simulink library "EdgesLibrary"  (R2021a)
settings: Solver=VariableStepAuto  StartTime=0.0  StopTime=10.0  RelTol=1e-3
undefined symbols (not defined in the file): Rk
libraries: $bdroot x11, simulink x5
settings Model: Creator=phill  LastModifiedBy=phill

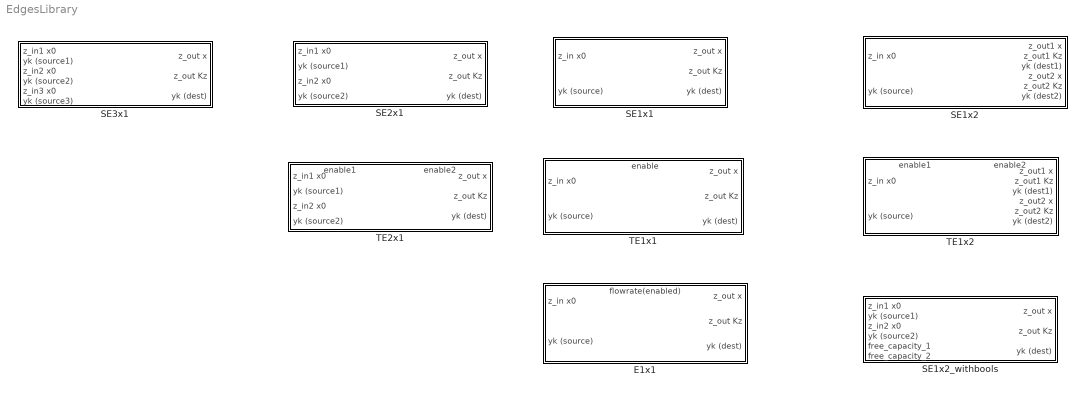
== system EdgesLibrary ==
  E1x1 : Subsystem
      mask help: This block serves to establish a flow between two Street Lane Segments. To archieve this, it connects one source-cell [z_in] to one destination-cell [z_out], and prompts a flow of cars with the flowrate 'flowrate(enabled)' (an input) if and only if there are still cars at the end of [z_out] avaiable AND if the capacity of [z_out] is not yet surpassed, i.e. (z_in x0 > 0 AND z_out Kz > z_out x), otherwise the flow is reduced to 0.
      settings: PortSchema="{\"entries\":[{\"content\":{\"sides\":[{\"content\":{\"connectorIds\":[\"In1\",\"Out2\"]},\"type\":\"ConnectorPlacement.EquallySpacedRectSide\",\"uuid\":\"c2e99070-5232-4a61-a40f-9294101b0b00\"},{\"content\":{\"connectorIds\":[\"In3\",\"In4\",\"Out1\"],\"side\":\"RIGHT\"},\"type\":\"ConnectorPlacement.EquallySpacedRectSide\",\"uuid\":\"7311a175-c780-45f4-b469-43cf69089bcd\"},{\"content\":{\"connectorIds\":[\"In2\"],\"side\":\"TOP\"},\"type\":\"ConnectorPlacement.EquallySpacedRectSide\",\"uuid\":\"52e907de-6c11-4251-aa6b-7e90a209cdcc\"}]},\"type\":\"ConnectorPlacement.EquallySpacedConnector\",\"uuid\":\"2a0e9608-1744-4ca6-8ee9-50c44ff0c1fb\"}],\"packageUris\":[\"http://schema.mathworks.com/mf0/Connector/R2020b\"],\"version\":\"1.0\"}"
      mask Display:
      | image('$imagefile'); % Use "Edit Image" on toolstrip to change.
      | % image('$imagefile');
      | disp('Edge 1x1');
  SE1x1 : Subsystem  mask{Rk=0, slope=2000}
      mask prompts: Rk "Rk (fixed flowrate, used when the flow is enabled)"
      mask help: This block serves to establish a flow between two Street Lane Segments. To archieve this, it connects one source-cell [z_in] to one destination-cell [z_out], and prompts a flow of cars with the rate Rk (Parameter) if and only if there are still cars at the end of [z_out] avaiable and if the capacity of [z_out] is not yet surpassed, i.e. (z_in x0 > 0 AND z_out Kz > z_out x), otherwise the flow is reduced to 0.
      settings: PortSchema="{\"entries\":[{\"content\":{\"sides\":[{\"content\":{\"connectorIds\":[\"In1\",\"Out2\"]},\"type\":\"ConnectorPlacement.EquallySpacedRectSide\",\"uuid\":\"f9c1cf46-46ac-4011-8499-7a2e74fc4a3a\"},{\"content\":{\"connectorIds\":[\"In2\",\"In3\",\"Out1\"],\"side\":\"RIGHT\"},\"type\":\"ConnectorPlacement.EquallySpacedRectSide\",\"uuid\":\"f685a77a-a8b9-4a29-8679-dc3cbf3c2b7f\"},{\"content\":{\"connectorIds\":[],\"side\":\"TOP\"},\"type\":\"ConnectorPlacement.EquallySpacedRectSide\",\"uuid\":\"af8d715a-ddb3-4f5e-8163-596be4e65ef7\"}]},\"type\":\"ConnectorPlacement.EquallySpacedConnector\",\"uuid\":\"ace495d2-b7cd-4153-a555-4989f077c969\"}],\"packageUris\":[\"http://schema.mathworks.com/mf0/Connector/R2020b\"],\"version\":\"1.0\"}"
      mask Display:
      | image('$imagefile'); % Use "Edit Image" on toolstrip to change.
      | % image('$imagefile');
      | disp('Simple Edge 1x1 \n\n');
      | disp(['Rk = ', get_param(gcb,'Rk'),' slope = ', get_param(gcb,'slope')])
  SE1x2 : Subsystem  mask{Rk1=0, Rk2=0}
      mask prompts: Rk1 "Rk (output 1)"; Rk2 "Rk (output 2)"
      settings: PortSchema="{\"entries\":[{\"content\":{\"sides\":[{\"content\":{\"connectorIds\":[\"In1\",\"Out3\"]},\"type\":\"ConnectorPlacement.EquallySpacedRectSide\",\"uuid\":\"58588114-80b7-4cf3-8a8f-92af49331a70\"},{\"content\":{\"connectorIds\":[\"In2\",\"In3\",\"Out1\",\"In4\",\"In5\",\"Out2\"],\"side\":\"RIGHT\"},\"type\":\"ConnectorPlacement.EquallySpacedRectSide\",\"uuid\":\"0e7c0143-84e4-4501-996a-3b666730c0e6\"},{\"content\":{\"connectorIds\":[],\"side\":\"TOP\"},\"type\":\"ConnectorPlacement.EquallySpacedRectSide\",\"uuid\":\"990b873b-8878-4c8e-bdf4-2f621fb88a1c\"}]},\"type\":\"ConnectorPlacement.EquallySpacedConnector\",\"uuid\":\"e53b41a9-82b8-4753-89eb-fe06ea1139d8\"}],\"packageUris\":[\"http://schema.mathworks.com/mf0/Connector/R2020b\"],\"version\":\"1.0\"}"
      mask Display:
      | image('$imagefile'); % Use "Edit Image" on toolstrip to change.
      | % image('$imagefile');
      | disp('Simple Edge 1x2\n\n\n');
      | tRk = get_param(gcb,'Rk1');
      | w1 = get_param(gcb, 'Rk2');
      | disp(['Rk1 = ', tRk, ' | Rk2 =  ', w1])
  SE1x2_withbools : Subsystem  mask{Rk1=Rk, Rk2=Rk}
      mask prompts: Rk1 "Rk (input 1)"; Rk2 "Rk (input 2)"
      settings: PortSchema="{\"entries\":[{\"content\":{\"sides\":[{\"content\":{\"connectorIds\":[\"In1\",\"Out2\",\"In2\",\"Out3\",\"Out4\",\"Out5\"]},\"type\":\"ConnectorPlacement.EquallySpacedRectSide\",\"uuid\":\"eb102e1f-8f68-4819-b192-9ed8ea7965cd\"},{\"content\":{\"connectorIds\":[\"In3\",\"In4\",\"Out1\"],\"side\":\"RIGHT\"},\"type\":\"ConnectorPlacement.EquallySpacedRectSide\",\"uuid\":\"0a8d41cc-2128-49e0-9ce9-20439c8bfca2\"},{\"content\":{\"connectorIds\":[],\"side\":\"TOP\"},\"type\":\"ConnectorPlacement.EquallySpacedRectSide\",\"uuid\":\"ce1e229b-7216-4f3c-b1ef-7720ca51f1c4\"}]},\"type\":\"ConnectorPlacement.EquallySpacedConnector\",\"uuid\":\"c8e8c67c-b38f-484f-95e7-011277152545\"}],\"packageUris\":[\"http://schema.mathworks.com/mf0/Connector/R2020b\"],\"version\":\"1.0\"}"
      mask Display:
      | image('$imagefile'); % Use "Edit Image" on toolstrip to change.
      | disp('Simple Edge 2x1\n\n\n');
      | Rk1 = get_param(gcb,'Rk1');
      | Rk2 = get_param(gcb, 'Rk2');
      | disp(['Rk1 = ', Rk1, ' | Rk2 =  ', Rk2])
  SE2x1 : Subsystem  mask{Rk1=0, Rk2=0}
      mask prompts: Rk1 "Rk (input 1)"; Rk2 "Rk (input 2)"
      settings: PortSchema="{\"entries\":[{\"content\":{\"sides\":[{\"content\":{\"connectorIds\":[\"In1\",\"Out2\",\"In2\",\"Out3\"]},\"type\":\"ConnectorPlacement.EquallySpacedRectSide\",\"uuid\":\"eb102e1f-8f68-4819-b192-9ed8ea7965cd\"},{\"content\":{\"connectorIds\":[\"In3\",\"In4\",\"Out1\"],\"side\":\"RIGHT\"},\"type\":\"ConnectorPlacement.EquallySpacedRectSide\",\"uuid\":\"0a8d41cc-2128-49e0-9ce9-20439c8bfca2\"},{\"content\":{\"connectorIds\":[],\"side\":\"TOP\"},\"type\":\"ConnectorPlacement.EquallySpacedRectSide\",\"uuid\":\"ce1e229b-7216-4f3c-b1ef-7720ca51f1c4\"}]},\"type\":\"ConnectorPlacement.EquallySpacedConnector\",\"uuid\":\"c8e8c67c-b38f-484f-95e7-011277152545\"}],\"packageUris\":[\"http://schema.mathworks.com/mf0/Connector/R2020b\"],\"version\":\"1.0\"}"
      mask Display:
      | image('$imagefile'); % Use "Edit Image" on toolstrip to change.
      | disp('Simple Edge 2x1\n\n\n');
      | Rk1 = get_param(gcb,'Rk1');
      | Rk2 = get_param(gcb, 'Rk2');
      | disp(['Rk1 = ', Rk1, ' | Rk2 =  ', Rk2])
  SE3x1 : Subsystem  mask{Rk1=0, Rk2=0, Rk3=0}
      mask prompts: Rk1 "Rk (input 1)"; Rk2 "Rk (input 2)"; Rk3 "Rk (input 3)"
      settings: PortSchema="{\"entries\":[{\"content\":{\"sides\":[{\"content\":{\"connectorIds\":[\"In1\",\"Out2\",\"In2\",\"Out3\",\"In3\",\"Out4\"]},\"type\":\"ConnectorPlacement.EquallySpacedRectSide\",\"uuid\":\"eb102e1f-8f68-4819-b192-9ed8ea7965cd\"},{\"content\":{\"connectorIds\":[\"In4\",\"In5\",\"Out1\"],\"side\":\"RIGHT\"},\"type\":\"ConnectorPlacement.EquallySpacedRectSide\",\"uuid\":\"0a8d41cc-2128-49e0-9ce9-20439c8bfca2\"},{\"content\":{\"connectorIds\":[],\"side\":\"TOP\"},\"type\":\"ConnectorPlacement.EquallySpacedRectSide\",\"uuid\":\"ce1e229b-7216-4f3c-b1ef-7720ca51f1c4\"}]},\"type\":\"ConnectorPlacement.EquallySpacedConnector\",\"uuid\":\"c8e8c67c-b38f-484f-95e7-011277152545\"}],\"packageUris\":[\"http://schema.mathworks.com/mf0/Connector/R2020b\"],\"version\":\"1.0\"}"
      mask Display:
      | image('$imagefile'); % Use "Edit Image" on toolstrip to change.
      | disp('Simple Edge 3x1\n\n\n');
      | Rk1 = get_param(gcb,'Rk1');
      | Rk2 = get_param(gcb, 'Rk2');
      | Rk3 = get_param(gcb, 'Rk3');
      | disp(['Rk1 = ', Rk1, ' | Rk2 =  ', Rk2, '\n | Rk3 = ', Rk3])
  TE1x1 : Subsystem  mask{Rk=0, slope=2000}
      mask prompts: Rk "Rk (fixed flowrate, used when the flow is enabled)"
      mask help: This block serves to establish a flow between two Street Lane Segments. To archieve this, it connects one source-cell [z_in] to one destination-cell [z_out], and prompts a flow of cars with the rate Rk (Parameter) if and only if there are still cars at the end of [z_out] avaiable AND if the capacity of [z_out] is not yet surpassed, i.e. (z_in x0 > 0 AND z_out Kz > z_out x), AND if the 'enable' input is set to 1, otherwise the flow is reduced to 0.
      settings: PortSchema="{\"entries\":[{\"content\":{\"sides\":[{\"content\":{\"connectorIds\":[\"In1\",\"Out2\"]},\"type\":\"ConnectorPlacement.EquallySpacedRectSide\",\"uuid\":\"c2e99070-5232-4a61-a40f-9294101b0b00\"},{\"content\":{\"connectorIds\":[\"In3\",\"In4\",\"Out1\"],\"side\":\"RIGHT\"},\"type\":\"ConnectorPlacement.EquallySpacedRectSide\",\"uuid\":\"7311a175-c780-45f4-b469-43cf69089bcd\"},{\"content\":{\"connectorIds\":[\"In2\"],\"side\":\"TOP\"},\"type\":\"ConnectorPlacement.EquallySpacedRectSide\",\"uuid\":\"52e907de-6c11-4251-aa6b-7e90a209cdcc\"}]},\"type\":\"ConnectorPlacement.EquallySpacedConnector\",\"uuid\":\"2a0e9608-1744-4ca6-8ee9-50c44ff0c1fb\"}],\"packageUris\":[\"http://schema.mathworks.com/mf0/Connector/R2020b\"],\"version\":\"1.0\"}"
      mask Display:
      | image('$imagefile'); % Use "Edit Image" on toolstrip to change.
      | % image('$imagefile');
      | disp('Toggleable Edge 1x1 \n\n');
      | disp(['Rk = ', get_param(gcb,'Rk'),' slope = ', get_param(gcb,'slope')])
  TE1x2 : Subsystem  mask{Rk1=0, Rk2=0}
      mask prompts: Rk1 "Rk (output 1)"; Rk2 "Rk (output 2)"
      settings: PortSchema="{\"entries\":[{\"content\":{\"sides\":[{\"content\":{\"connectorIds\":[\"In1\",\"Out3\"]},\"type\":\"ConnectorPlacement.EquallySpacedRectSide\",\"uuid\":\"2e9f11d3-65d9-473f-b826-57e0db4d0b8d\"},{\"content\":{\"connectorIds\":[\"In4\",\"In5\",\"Out1\",\"In6\",\"In7\",\"Out2\"],\"side\":\"RIGHT\"},\"type\":\"ConnectorPlacement.EquallySpacedRectSide\",\"uuid\":\"d8eabf6d-fb3a-4c3e-97ce-4f99fedc7242\"},{\"content\":{\"connectorIds\":[\"In2\",\"In3\"],\"side\":\"TOP\"},\"type\":\"ConnectorPlacement.EquallySpacedRectSide\",\"uuid\":\"c1317a9d-7aa4-490c-a27e-f3fa93a0d151\"}]},\"type\":\"ConnectorPlacement.EquallySpacedConnector\",\"uuid\":\"3cd892e4-da09-4624-b831-53c46896b420\"}],\"packageUris\":[\"http://schema.mathworks.com/mf0/Connector/R2020b\"],\"version\":\"1.0\"}"
      mask Display:
      | image('$imagefile'); % Use "Edit Image" on toolstrip to change.
      | disp('Toggleable Edge 1x2 \n\n');
      | Rk1 = get_param(gcb,'Rk1');
      | Rk2 = get_param(gcb, 'Rk2');
      | disp(['Rk1 = ', Rk1, ' | Rk2 =  ', Rk2])
  TE2x1 : Subsystem  mask{Rk1=0, Rk2=0.5}
      mask prompts: Rk1 "Rk (input 1)"; Rk2 "Rk (input 2)"
      settings: PortSchema="{\"entries\":[{\"content\":{\"sides\":[{\"content\":{\"connectorIds\":[\"In1\",\"Out2\",\"In2\",\"Out3\"]},\"type\":\"ConnectorPlacement.EquallySpacedRectSide\",\"uuid\":\"2e9f11d3-65d9-473f-b826-57e0db4d0b8d\"},{\"content\":{\"connectorIds\":[\"In5\",\"In6\",\"Out1\"],\"side\":\"RIGHT\"},\"type\":\"ConnectorPlacement.EquallySpacedRectSide\",\"uuid\":\"d8eabf6d-fb3a-4c3e-97ce-4f99fedc7242\"},{\"content\":{\"connectorIds\":[\"In3\",\"In4\"],\"side\":\"TOP\"},\"type\":\"ConnectorPlacement.EquallySpacedRectSide\",\"uuid\":\"c1317a9d-7aa4-490c-a27e-f3fa93a0d151\"}]},\"type\":\"ConnectorPlacement.EquallySpacedConnector\",\"uuid\":\"3cd892e4-da09-4624-b831-53c46896b420\"}],\"packageUris\":[\"http://schema.mathworks.com/mf0/Connector/R2020b\"],\"version\":\"1.0\"}"
      mask Display:
      | image('$imagefile'); % Use "Edit Image" on toolstrip to change.
      | disp('Toggleable Edge 2x1 \n\n');
      | Rk1 = get_param(gcb,'Rk1');
      | Rk2 = get_param(gcb, 'Rk2');
      | disp(['Rk1 = ', Rk1, ' | Rk2 =  ', Rk2])

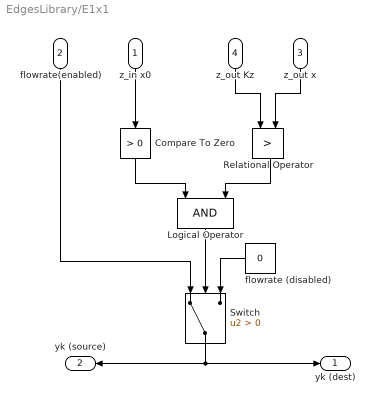
== system EdgesLibrary/E1x1 ==
  z_in x0 : Inport
  flowrate(enabled) : Inport  Port=2
  z_out x : Inport  Port=3
  z_out Kz : Inport  Port=4
  Compare To Zero : simulink/Logic and Bit Operations/Compare To Zero  relop=>  OutDataTypeStr=boolean
  Logical Operator : Logic  Inputs=3  AllPortsSameDT=off  OutDataTypeStr=boolean
  Relational Operator : RelationalOperator  Operator=>  OutDataTypeStr=boolean  RndMeth=Simplest
  Switch : Switch  Criteria=u2 > Threshold
  flowrate (disabled) : Constant  Value=0
  yk (dest) : Outport
  yk (source) : Outport  Port=2
  wires:
  z_out Kz/1 -> Relational Operator/1
  z_out x/1 -> Relational Operator/2
  Logical Operator/1 -> Switch/2
  flowrate(enabled)/1 -> Switch/1
  flowrate (disabled)/1 -> Switch/3
  z_in x0/1 -> Compare To Zero/1
  Compare To Zero/1 -> Logical Operator/1
  Relational Operator/1 -> Logical Operator/3
  Switch/1 -> yk (source)/1, yk (dest)/1

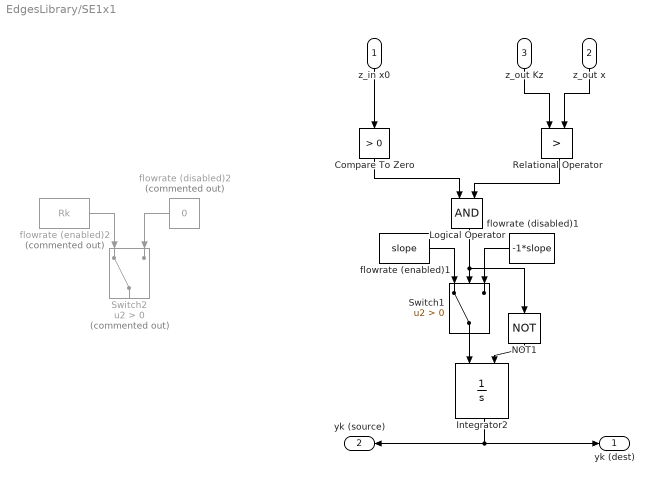
== system EdgesLibrary/SE1x1 ==
  z_in x0 : Inport
  z_out x : Inport  Port=2
  z_out Kz : Inport  Port=3
  Compare To Zero : simulink/Logic and Bit Operations/Compare To Zero  relop=>  OutDataTypeStr=boolean
  Integrator2 : Integrator  ExternalReset=rising  LimitOutput=on  UpperSaturationLimit=Rk  LowerSaturationLimit=0
  Logical Operator : Logic  AllPortsSameDT=off  OutDataTypeStr=boolean
  NOT1 : Logic  Operator=NOT  IconShape=distinctive  AllPortsSameDT=off  OutDataTypeStr=boolean
  Relational Operator : RelationalOperator  Operator=>  OutDataTypeStr=boolean  RndMeth=Simplest
  Switch1 : Switch  Criteria=u2 > Threshold
  Switch2 : Switch  Commented=on  Criteria=u2 > Threshold
  flowrate (disabled)1 : Constant  Value=-1*slope
  flowrate (disabled)2 : Constant  Commented=on  Value=0
  flowrate (enabled)1 : Constant  Value=slope
  flowrate (enabled)2 : Constant  Commented=on  Value=Rk
  yk (dest) : Outport
  yk (source) : Outport  Port=2
  wires:
  Compare To Zero/1 -> Logical Operator/1
  z_out x/1 -> Relational Operator/2
  z_out Kz/1 -> Relational Operator/1
  Integrator2/1 -> yk (source)/1, yk (dest)/1
  Relational Operator/1 -> Logical Operator/2
  z_in x0/1 -> Compare To Zero/1
  flowrate (enabled)1/1 -> Switch1/1
  Switch1/1 -> Integrator2/1
  Logical Operator/1 -> NOT1/1, Switch1/2
  NOT1/1 -> Integrator2/2
  flowrate (disabled)1/1 -> Switch1/3
  flowrate (disabled)2/1 -> Switch2/3
  flowrate (enabled)2/1 -> Switch2/1
  ? -> Switch2/2

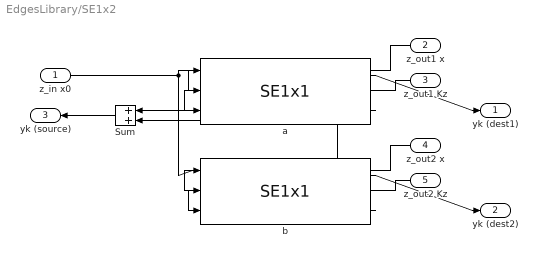
== system EdgesLibrary/SE1x2 ==
  z_in x0 : Inport
  z_out1 x : Inport  Port=2
  z_out1 Kz : Inport  Port=3
  z_out2 x : Inport  Port=4
  z_out2 Kz : Inport  Port=5
  Sum : Sum
  a : $bdroot/SE1x1  Rk=Rk1  slope=2000
  b : $bdroot/SE1x1  Rk=Rk2  slope=2000
  yk (dest1) : Outport
  yk (dest2) : Outport  Port=2
  yk (source) : Outport  Port=3
  wires:
  z_out1 x/1 -> a/2
  z_out1 Kz/1 -> a/3
  z_out2 Kz/1 -> b/3
  z_out2 x/1 -> b/2
  a/2 -> Sum/1
  b/2 -> Sum/2
  Sum/1 -> yk (source)/1
  b/1 -> yk (dest2)/1
  a/1 -> yk (dest1)/1
  z_in x0/1 -> b/1, a/1

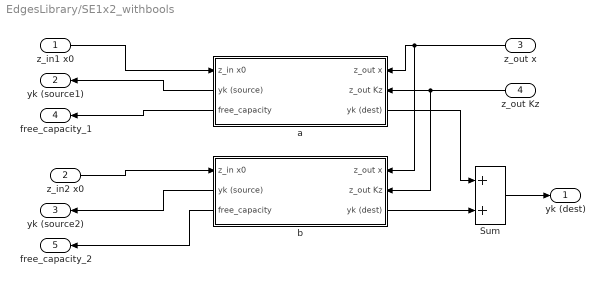
== system EdgesLibrary/SE1x2_withbools ==
  z_in1 x0 : Inport
  z_in2 x0 : Inport  Port=2
  z_out x : Inport  Port=3
  z_out Kz : Inport  Port=4
  Sum : Sum
  a : Subsystem  mask{Rk=Rk1, slope=2000}
      mask prompts: Rk "Rk (fixed flowrate, used when the flow is enabled)"
      mask help: This block serves to establish a flow between two Street Lane Segments. To archieve this, it connects one source-cell [z_in] to one destination-cell [z_out], and prompts a flow of cars with the rate Rk (Parameter) if and only if there are still cars at the end of [z_out] avaiable and if the capacity of [z_out] is not yet surpassed, i.e. (z_in x0 > 0 AND z_out Kz > z_out x), otherwise the flow is reduced to 0.
      settings: PortSchema="{\"entries\":[{\"content\":{\"sides\":[{\"content\":{\"connectorIds\":[\"In1\",\"Out2\",\"Out3\"]},\"type\":\"ConnectorPlacement.EquallySpacedRectSide\",\"uuid\":\"f9c1cf46-46ac-4011-8499-7a2e74fc4a3a\"},{\"content\":{\"connectorIds\":[\"In2\",\"In3\",\"Out1\"],\"side\":\"RIGHT\"},\"type\":\"ConnectorPlacement.EquallySpacedRectSide\",\"uuid\":\"f685a77a-a8b9-4a29-8679-dc3cbf3c2b7f\"},{\"content\":{\"connectorIds\":[],\"side\":\"TOP\"},\"type\":\"ConnectorPlacement.EquallySpacedRectSide\",\"uuid\":\"af8d715a-ddb3-4f5e-8163-596be4e65ef7\"}]},\"type\":\"ConnectorPlacement.EquallySpacedConnector\",\"uuid\":\"ace495d2-b7cd-4153-a555-4989f077c969\"}],\"packageUris\":[\"http://schema.mathworks.com/mf0/Connector/R2020b\"],\"version\":\"1.0\"}"
      mask Display:
      | image('$imagefile'); % Use "Edit Image" on toolstrip to change.
      | % image('$imagefile');
      | disp('Simple Edge 1x1 \n\n');
      | disp(['Rk = ', get_param(gcb,'Rk'),' slope = ', get_param(gcb,'slope')])
  b : Subsystem  mask{Rk=Rk2, slope=2000}
      mask prompts: Rk "Rk (fixed flowrate, used when the flow is enabled)"
      mask help: This block serves to establish a flow between two Street Lane Segments. To archieve this, it connects one source-cell [z_in] to one destination-cell [z_out], and prompts a flow of cars with the rate Rk (Parameter) if and only if there are still cars at the end of [z_out] avaiable and if the capacity of [z_out] is not yet surpassed, i.e. (z_in x0 > 0 AND z_out Kz > z_out x), otherwise the flow is reduced to 0.
      settings: PortSchema="{\"entries\":[{\"content\":{\"sides\":[{\"content\":{\"connectorIds\":[\"In1\",\"Out2\",\"Out3\"]},\"type\":\"ConnectorPlacement.EquallySpacedRectSide\",\"uuid\":\"f9c1cf46-46ac-4011-8499-7a2e74fc4a3a\"},{\"content\":{\"connectorIds\":[\"In2\",\"In3\",\"Out1\"],\"side\":\"RIGHT\"},\"type\":\"ConnectorPlacement.EquallySpacedRectSide\",\"uuid\":\"f685a77a-a8b9-4a29-8679-dc3cbf3c2b7f\"},{\"content\":{\"connectorIds\":[],\"side\":\"TOP\"},\"type\":\"ConnectorPlacement.EquallySpacedRectSide\",\"uuid\":\"af8d715a-ddb3-4f5e-8163-596be4e65ef7\"}]},\"type\":\"ConnectorPlacement.EquallySpacedConnector\",\"uuid\":\"ace495d2-b7cd-4153-a555-4989f077c969\"}],\"packageUris\":[\"http://schema.mathworks.com/mf0/Connector/R2020b\"],\"version\":\"1.0\"}"
      mask Display:
      | image('$imagefile'); % Use "Edit Image" on toolstrip to change.
      | % image('$imagefile');
      | disp('Simple Edge 1x1 \n\n');
      | disp(['Rk = ', get_param(gcb,'Rk'),' slope = ', get_param(gcb,'slope')])
  yk (dest) : Outport
  yk (source1) : Outport  Port=2
  yk (source2) : Outport  Port=3
  free_capacity_1 : Outport  Port=4
  free_capacity_2 : Outport  Port=5
  wires:
  z_out Kz/1 -> b/3(z_out Kz), a/3(z_out Kz)
  Sum/1 -> yk (dest)/1
  z_out x/1 -> b/2(z_out x), a/2(z_out x)
  b/1(yk (dest)) -> Sum/2
  z_in1 x0/1 -> a/1(z_in x0)
  a/1(yk (dest)) -> Sum/1
  z_in2 x0/1 -> b/1(z_in x0)
  b/2(yk (source)) -> yk (source2)/1
  a/2(yk (source)) -> yk (source1)/1
  a/3(free_capacity) -> free_capacity_1/1
  b/3(free_capacity) -> free_capacity_2/1

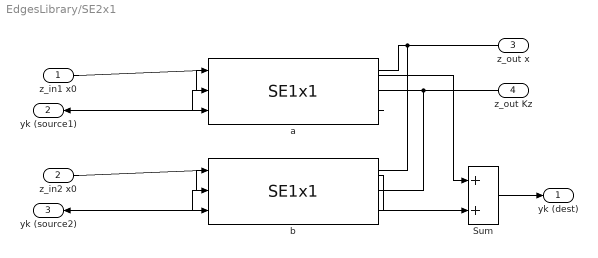
== system EdgesLibrary/SE2x1 ==
  z_in1 x0 : Inport
  z_in2 x0 : Inport  Port=2
  z_out x : Inport  Port=3
  z_out Kz : Inport  Port=4
  Sum : Sum
  a : $bdroot/SE1x1  Rk=Rk1
  b : $bdroot/SE1x1  Rk=Rk2
  yk (dest) : Outport
  yk (source1) : Outport  Port=2
  yk (source2) : Outport  Port=3
  wires:
  a/2 -> yk (source1)/1
  b/2 -> yk (source2)/1
  z_in2 x0/1 -> b/1
  a/1 -> Sum/1
  z_in1 x0/1 -> a/1
  b/1 -> Sum/2
  z_out x/1 -> a/2, b/2
  Sum/1 -> yk (dest)/1
  z_out Kz/1 -> a/3, b/3

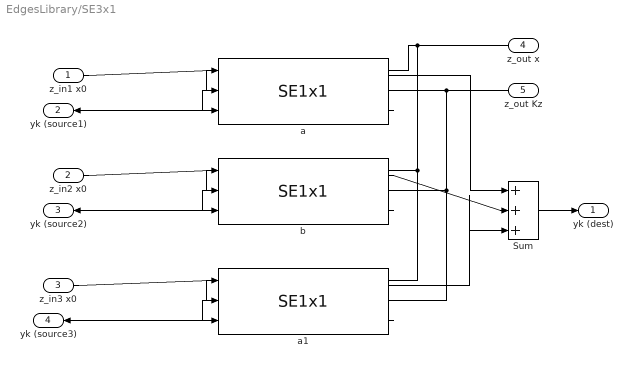
== system EdgesLibrary/SE3x1 ==
  z_in1 x0 : Inport
  z_in2 x0 : Inport  Port=2
  z_in3 x0 : Inport  Port=3
  z_out x : Inport  Port=4
  z_out Kz : Inport  Port=5
  Sum : Sum  Inputs=+++
  a : $bdroot/SE1x1  Rk=Rk1  slope=200
  a1 : $bdroot/SE1x1  Rk=Rk3  slope=200
  b : $bdroot/SE1x1  Rk=Rk2  slope=200
  yk (dest) : Outport
  yk (source1) : Outport  Port=2
  yk (source2) : Outport  Port=3
  yk (source3) : Outport  Port=4
  wires:
  a/2 -> yk (source1)/1
  b/2 -> yk (source2)/1
  z_in2 x0/1 -> b/1
  a/1 -> Sum/1
  z_in1 x0/1 -> a/1
  b/1 -> Sum/2
  z_out x/1 -> a/2, a1/2, b/2
  Sum/1 -> yk (dest)/1
  z_out Kz/1 -> a/3, b/3, a1/3
  z_in3 x0/1 -> a1/1
  a1/2 -> yk (source3)/1
  a1/1 -> Sum/3

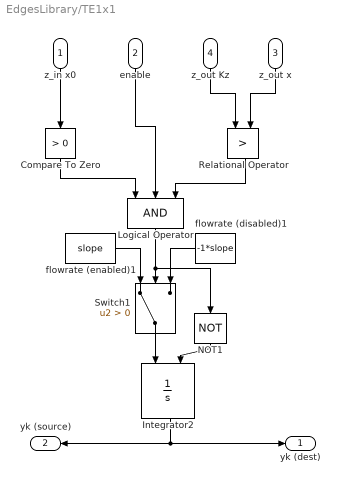
== system EdgesLibrary/TE1x1 ==
  z_in x0 : Inport
  enable : Inport  Port=2
  z_out x : Inport  Port=3
  z_out Kz : Inport  Port=4
  Compare To Zero : simulink/Logic and Bit Operations/Compare To Zero  relop=>  OutDataTypeStr=boolean
  Integrator2 : Integrator  ExternalReset=rising  LimitOutput=on  UpperSaturationLimit=Rk  LowerSaturationLimit=0
  Logical Operator : Logic  Inputs=3  AllPortsSameDT=off  OutDataTypeStr=boolean
  NOT1 : Logic  Operator=NOT  IconShape=distinctive  AllPortsSameDT=off  OutDataTypeStr=boolean
  Relational Operator : RelationalOperator  Operator=>  OutDataTypeStr=boolean  RndMeth=Simplest
  Switch1 : Switch  Criteria=u2 > Threshold
  flowrate (disabled)1 : Constant  Value=-1*slope
  flowrate (enabled)1 : Constant  Value=slope
  yk (dest) : Outport
  yk (source) : Outport  Port=2
  wires:
  z_out Kz/1 -> Relational Operator/1
  enable/1 -> Logical Operator/2
  Compare To Zero/1 -> Logical Operator/1
  Integrator2/1 -> yk (source)/1, yk (dest)/1
  Relational Operator/1 -> Logical Operator/3
  z_out x/1 -> Relational Operator/2
  z_in x0/1 -> Compare To Zero/1
  flowrate (disabled)1/1 -> Switch1/3
  Switch1/1 -> Integrator2/1
  NOT1/1 -> Integrator2/2
  flowrate (enabled)1/1 -> Switch1/1
  Logical Operator/1 -> NOT1/1, Switch1/2

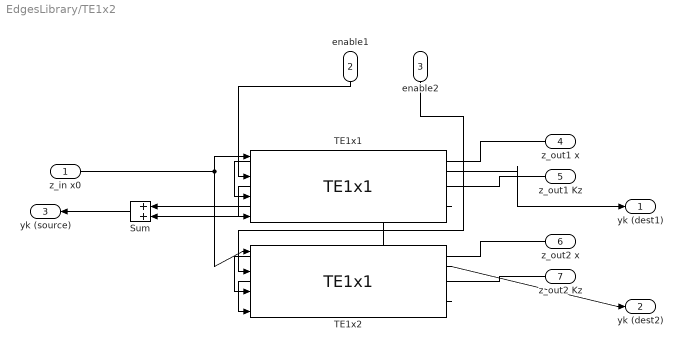
== system EdgesLibrary/TE1x2 ==
  z_in x0 : Inport
  enable1 : Inport  Port=2
  enable2 : Inport  Port=3
  z_out1 x : Inport  Port=4
  z_out1 Kz : Inport  Port=5
  z_out2 x : Inport  Port=6
  z_out2 Kz : Inport  Port=7
  Sum : Sum
  TE1x1 : $bdroot/TE1x1  Rk=Rk1  slope=2000
  TE1x2 : $bdroot/TE1x1  Rk=Rk2  slope=2000
  yk (dest1) : Outport
  yk (dest2) : Outport  Port=2
  yk (source) : Outport  Port=3
  wires:
  enable2/1 -> TE1x2/2
  z_out2 x/1 -> TE1x2/3
  Sum/1 -> yk (source)/1
  TE1x1/2 -> Sum/1
  z_in x0/1 -> TE1x1/1, TE1x2/1
  z_out2 Kz/1 -> TE1x2/4
  TE1x2/2 -> Sum/2
  TE1x2/1 -> yk (dest2)/1
  z_out1 Kz/1 -> TE1x1/4
  z_out1 x/1 -> TE1x1/3
  enable1/1 -> TE1x1/2
  TE1x1/1 -> yk (dest1)/1

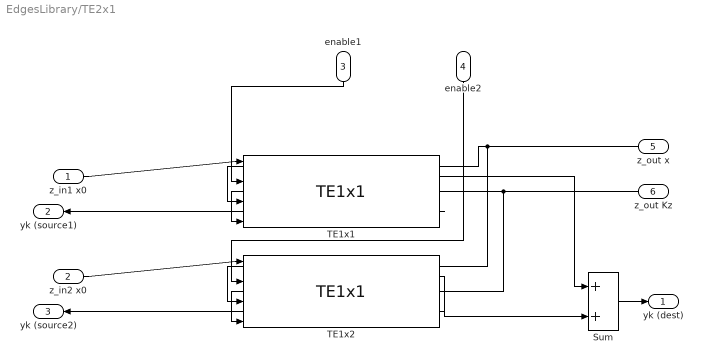
== system EdgesLibrary/TE2x1 ==
  z_in1 x0 : Inport
  z_in2 x0 : Inport  Port=2
  enable1 : Inport  Port=3
  enable2 : Inport  Port=4
  z_out x : Inport  Port=5
  z_out Kz : Inport  Port=6
  Sum : Sum
  TE1x1 : $bdroot/TE1x1  Rk=Rk1
  TE1x2 : $bdroot/TE1x1  Rk=Rk2
  yk (dest) : Outport
  yk (source1) : Outport  Port=2
  yk (source2) : Outport  Port=3
  wires:
  TE1x1/2 -> yk (source1)/1
  z_in1 x0/1 -> TE1x1/1
  TE1x2/2 -> yk (source2)/1
  enable1/1 -> TE1x1/2
  enable2/1 -> TE1x2/2
  TE1x1/1 -> Sum/1
  z_out Kz/1 -> TE1x2/4, TE1x1/4
  z_in2 x0/1 -> TE1x2/1
  TE1x2/1 -> Sum/2
  z_out x/1 -> TE1x2/3, TE1x1/3
  Sum/1 -> yk (dest)/1

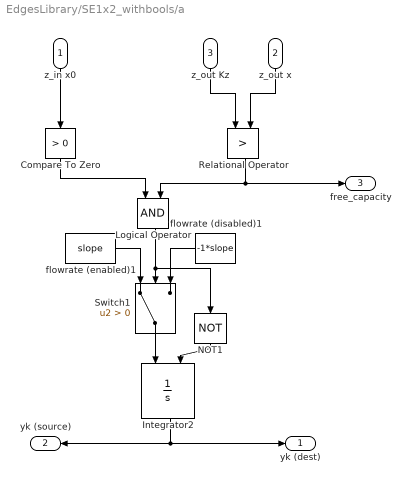
== system EdgesLibrary/SE1x2_withbools/a ==
  z_in x0 : Inport
  z_out x : Inport  Port=2
  z_out Kz : Inport  Port=3
  Compare To Zero : simulink/Logic and Bit Operations/Compare To Zero  relop=>  OutDataTypeStr=boolean
  Integrator2 : Integrator  ExternalReset=rising  LimitOutput=on  UpperSaturationLimit=Rk  LowerSaturationLimit=0
  Logical Operator : Logic  AllPortsSameDT=off  OutDataTypeStr=boolean
  NOT1 : Logic  Operator=NOT  IconShape=distinctive  AllPortsSameDT=off  OutDataTypeStr=boolean
  Relational Operator : RelationalOperator  Operator=>  OutDataTypeStr=boolean  RndMeth=Simplest
  Switch1 : Switch  Criteria=u2 > Threshold
  flowrate (disabled)1 : Constant  Value=-1*slope
  flowrate (enabled)1 : Constant  Value=slope
  yk (dest) : Outport
  yk (source) : Outport  Port=2
  free_capacity : Outport  Port=3
  wires:
  z_in x0/1 -> Compare To Zero/1
  Integrator2/1 -> yk (dest)/1, yk (source)/1
  z_out Kz/1 -> Relational Operator/1
  z_out x/1 -> Relational Operator/2
  Compare To Zero/1 -> Logical Operator/1
  Relational Operator/1 -> Logical Operator/2, free_capacity/1
  flowrate (disabled)1/1 -> Switch1/3
  Switch1/1 -> Integrator2/1
  NOT1/1 -> Integrator2/2
  flowrate (enabled)1/1 -> Switch1/1
  Logical Operator/1 -> NOT1/1, Switch1/2

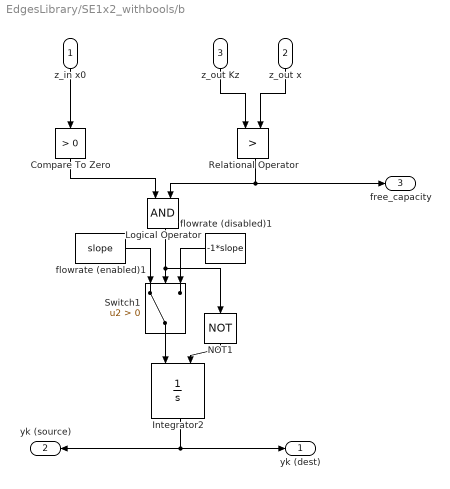
== system EdgesLibrary/SE1x2_withbools/b ==
  z_in x0 : Inport
  z_out x : Inport  Port=2
  z_out Kz : Inport  Port=3
  Compare To Zero : simulink/Logic and Bit Operations/Compare To Zero  relop=>  OutDataTypeStr=boolean
  Integrator2 : Integrator  ExternalReset=rising  LimitOutput=on  UpperSaturationLimit=Rk  LowerSaturationLimit=0
  Logical Operator : Logic  AllPortsSameDT=off  OutDataTypeStr=boolean
  NOT1 : Logic  Operator=NOT  IconShape=distinctive  AllPortsSameDT=off  OutDataTypeStr=boolean
  Relational Operator : RelationalOperator  Operator=>  OutDataTypeStr=boolean  RndMeth=Simplest
  Switch1 : Switch  Criteria=u2 > Threshold
  flowrate (disabled)1 : Constant  Value=-1*slope
  flowrate (enabled)1 : Constant  Value=slope
  yk (dest) : Outport
  yk (source) : Outport  Port=2
  free_capacity : Outport  Port=3
  wires:
  z_in x0/1 -> Compare To Zero/1
  Integrator2/1 -> yk (source)/1, yk (dest)/1
  z_out Kz/1 -> Relational Operator/1
  z_out x/1 -> Relational Operator/2
  Compare To Zero/1 -> Logical Operator/1
  Relational Operator/1 -> free_capacity/1, Logical Operator/2
  flowrate (disabled)1/1 -> Switch1/3
  Switch1/1 -> Integrator2/1
  NOT1/1 -> Integrator2/2
  flowrate (enabled)1/1 -> Switch1/1
  Logical Operator/1 -> NOT1/1, Switch1/2
